simulink model "lab4_1"  (R2023a)
settings: Solver=VariableStepAuto  StartTime=0.0  StopTime=10.0  RelTol=1e-3
undefined symbols (not defined in the file or in its folder): C, Ce, Le, u0, x0
libraries: simulink x1
settings Model: Creator=bz  LastModifiedBy=bz

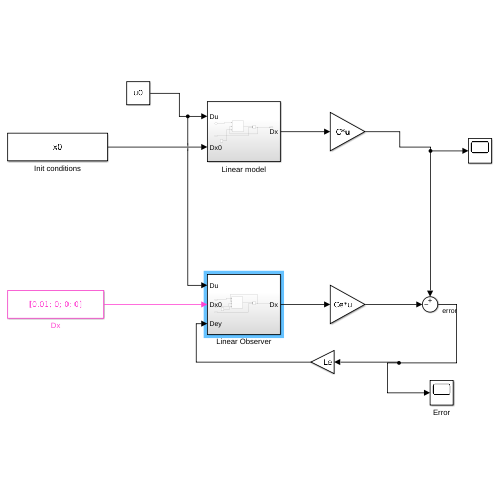
[thumbnail: Simulink's stored preview of the top-level diagram]
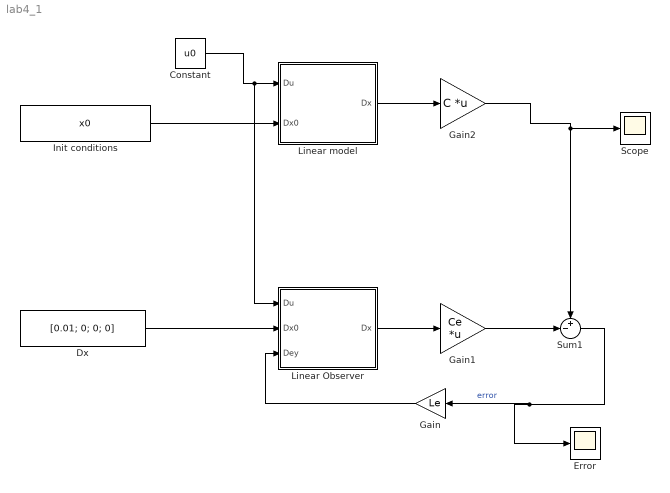
== system lab4_1 ==
  Constant : Constant  Value=u0
  Dx : Constant  Value=[0.01; 0; 0; 0]  VectorParams1D=off
  Error : Scope
  Gain : Gain  Gain=Le
  Gain1 : Gain  Gain=Ce  Multiplication=Matrix(K*u)
  Gain2 : Gain  Gain=C  Multiplication=Matrix(K*u)
  Init conditions : Constant  Value=x0  VectorParams1D=off
  Linear Observer : Subsystem
  Linear model : Subsystem
  Scope : Scope
  Sum1 : Sum  Inputs=+-|
  wires:
  Init conditions/1 -> Linear model/2(Dx0)
  Dx/1 -> Linear Observer/2(Dx0)
  Linear Observer/1(Dx) -> Gain1/1
  Gain1/1 -> Sum1/2
  Linear model/1(Dx) -> Gain2/1
  Gain2/1 -> Scope/1, Sum1/1
  Sum1/1 -> Gain/1, Error/1  "error"
  Gain/1 -> Linear Observer/3(Dey)
  Constant/1 -> Linear Observer/1(Du), Linear model/1(Du)

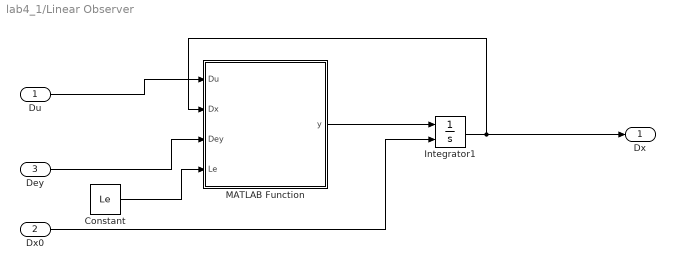
== system lab4_1/Linear Observer ==
  Du : Inport
  Dx0 : Inport  Port=2
  Dey : Inport  Port=3
  Constant : Constant  Value=Le
  Integrator1 : Integrator  InitialConditionSource=external
  MATLAB Function : MATLAB Function  TreatAsAtomicUnit=on
  Dx : Outport
  wires:
  MATLAB Function/1(y) -> Integrator1/1
  Dx0/1 -> Integrator1/2
  Integrator1/1 -> MATLAB Function/2(Dx), Dx/1
  Du/1 -> MATLAB Function/1(Du)
  Dey/1 -> MATLAB Function/3(Dey)
  Constant/1 -> MATLAB Function/4(Le)

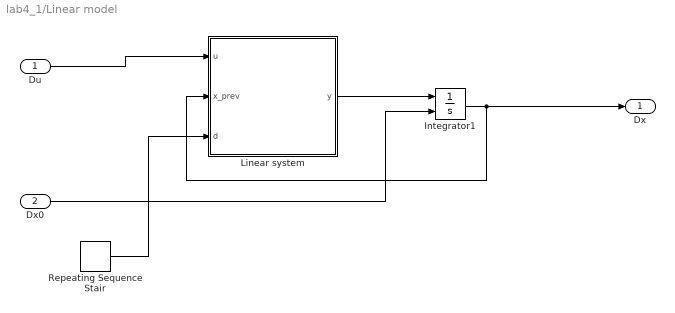
== system lab4_1/Linear model ==
  Du : Inport
  Dx0 : Inport  Port=2
  Integrator1 : Integrator  InitialConditionSource=external
  Linear system : MATLAB Function  TreatAsAtomicUnit=on
  Repeating Sequence Stair : simulink/Sources/Repeating Sequence Stair  OutValues=[5 1 2 2 1].'  tsamp=10  OutMin=[]  OutMax=[]  OutDataTypeStr=double  OutputDataTypeScalingMode=double  OutDataType=fixdt(0,8)  ConRadixGroup=Best Precision: Vector-wise  OutScaling=2^-12
  Dx : Outport
  wires:
  Linear system/1(y) -> Integrator1/1
  Dx0/1 -> Integrator1/2
  Integrator1/1 -> Dx/1, Linear system/2(x_prev)
  Du/1 -> Linear system/1(u)
  Repeating Sequence Stair/1 -> Linear system/3(d)

== matlab function lab4_1/Linear model/Linear system ==
  data: u input; y output size=[3,1]; x_prev input; d input
function y  = fcn(u, x_prev, d)

A = [0              0.0010      0;
     1.6847         0           -0.0257;
     0              0           -0.2888] * 1e3;

B = [0;
     0;
     1.2706] * 1e3;

E =[
    1;
    0;
    0
];

y = A * x_prev + B * u + E * d;

end

== matlab function lab4_1/Linear Observer/MATLAB Function ==
  data: Du input; y output; Dx input; Dey input; Le input
function y  = observer(Du, Dx, Dey, Le)

A = [0              0.0010      0;
     1.6847         0           -0.0257;
     0              0           -0.2888] * 1e3;

E = [1; 0; 0];

Ae = [A E;
     zeros(1, 4)];

B = [0;
     0;
     1.2706] * 1e3;

Be = [B; 0];

y = Ae * Dx + Be * Du + Le .* Dey;
% y = zeros(4,1);
end
